simulink model "simulink_template_2_3_base"  (R2024b)
settings: Solver=FixedStepAuto  StartTime=0.0  StopTime=10.0  FixedStep=1e-3  RelTol=1e-3
values from neighbouring files (symbols this model uses):
  a = vc/Ta    (= 0.333333333333)    [fcn.m]    (also in part2.m = [xf,xi,kf*cos(thetaf)-3*xf, ki*cos(thetai)+3*xi ])
  b = [yf,yi,kf*sin(thetaf)-3*yf, ki*sin(thetai)+3*yi ]    [part2.m]
  qi = [-1; -1; pi/2]    [EX_opt_2_leo.m]    (also in part2.m = [xi;yi;thetai]; script_2_motion_planning.m)
settings Model: Creator=alber  LastModifiedBy=loren
settings RTWCC: GPUComputeCapability=3.5

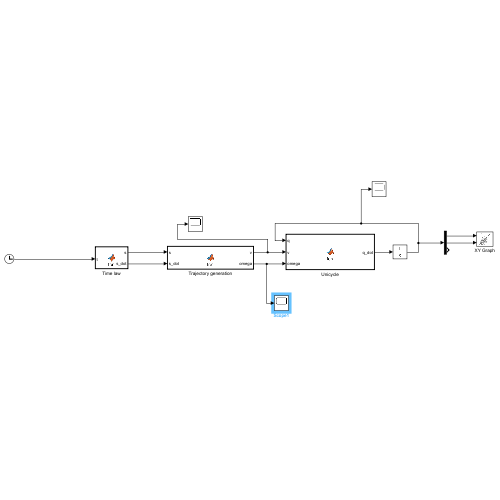
[thumbnail: Simulink's stored preview of the top-level diagram]
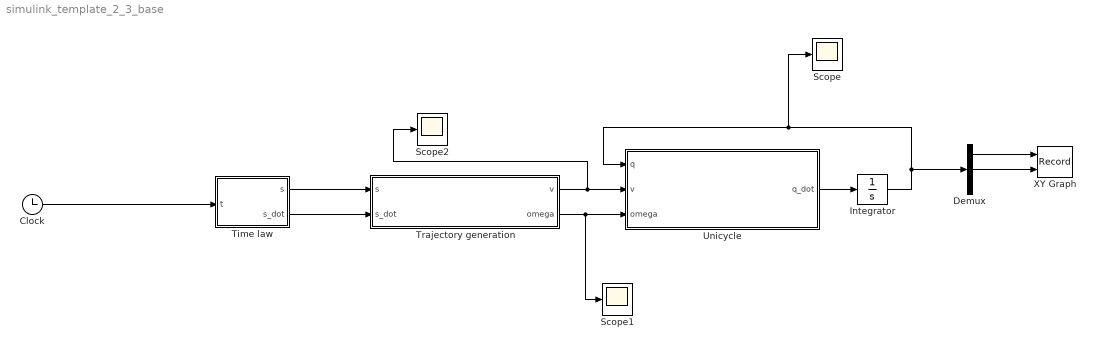
== system simulink_template_2_3_base ==
  Clock : Clock
  Demux : Demux  Outputs=3
  Integrator : Integrator  InitialCondition=qi
  Scope : Scope
  Scope1 : Scope
  Scope2 : Scope
  Time law : MATLAB Function  TreatAsAtomicUnit=on
  Trajectory generation : MATLAB Function  TreatAsAtomicUnit=on
  Unicycle : MATLAB Function  TreatAsAtomicUnit=on
  XY Graph : Record  FileSettingsInternal="{\"entries\":[{\"content\":{\"excelSettings\":{\"content\":{},\"type\":\"Streamout.ExcelSettings\"}},\"type\":\"Streamout.FileSettingStorage\",\"uuid\":\"\"}],\"packageUris\":[\"http:\\/\\/schema.mathworks.com\\/mf0\\/streamout_blocks\\/R2020a\"],\"version\":\"1.0\"}"  Layout=[1 1]  SignalsInternal="{\"entries\":[{\"content\":{\"signals\":[{\"content\":{\"blockPath\":[],\"dimensions\":[1,1],\"domain\":\"\",\"lineColor\":\"#a2142f\",\"lineWidth\":2,\"port\":1,\"sid\":[\"\"],\"signalID\":1,\"signalName\":\"Demux:1\"},\"type\":\"RecordBlkView.Signal\",\"uuid\":\"\"},{\"content\":{\"blockPath\":[],\"dimensions\":[1,1],\"domain\":\"\",\"lineColor\":\"#139fff\",\"plots\":[ 1 ],\"port\":2,\"sid\":[\"\"],\"signalID\":2,\"signalName\":\"Demux:2\"},\"type\":\"RecordBlkView.Signal\",\"uuid\":\"\"}]},\"type\":\"RecordBlkView.InputSignals\",\"uuid\":\"\"}],\"packageUris\":[\"http:\\/\\/schema.mathworks.com\\/mf0\\/streamout_blocks\\/R2020a\"],\"version\":\"1.0\"}"  VisualizationBindings="{\"xyplotplugin\":{\"info\":[{\"series\":[{\"bindingParametersList\":[{\"parameter\":\"Y-Axis\",\"signalID\":2,\"signalName\":\"Demux:2\"}],\"seriesID\":0}],\"subplotID\":1}]}}"  CompatibilityTag=XY
  wires:
  Clock/1 -> Time law/1(t)
  Time law/1(s) -> Trajectory generation/1(s)
  Time law/2(s_dot) -> Trajectory generation/2(s_dot)
  Trajectory generation/1(v) -> Scope2/1, Unicycle/2(v)
  Trajectory generation/2(omega) -> Scope1/1, Unicycle/3(omega)
  Unicycle/1(q_dot) -> Integrator/1
  Integrator/1 -> Scope/1, Unicycle/1(q), Demux/1
  Demux/1 -> XY Graph/1
  Demux/2 -> XY Graph/2

== matlab function simulink_template_2_3_base/Trajectory generation ==
  data: v output; s input; s_dot input; omega output; a parameter; b parameter
function [v, omega] = fcn(s, s_dot, a, b)
    % 1. Calcolo delle derivate spaziali prime (x' e y')
    % Basate sul polinomio cubico: y1(s) = a1*s^3 - a2*(s-1)^3 + a3*s^2*(s-1) + a4*s*(s-1)^2
    x_p = 3*a(1)*s^2 - a(2)*(3*s^2 - 6*s + 3) + a(3)*(3*s^2 - 2*s) + a(4)*(3*s^2 - 4*s + 1);
    y_p = 3*b(1)*s^2 - b(2)*(3*s^2 - 6*s + 3) + b(3)*(3*s^2 - 2*s) + b(4)*(3*s^2 - 4*s + 1);
    
    % 2. Calcolo delle derivate spaziali seconde (x'' e y'')
    x_pp = 6*a(1)*s - a(2)*(6*s - 6) + a(3)*(6*s - 2) + a(4)*(6*s - 4);
    y_pp = 6*b(1)*s - b(2)*(6*s - 6) + b(3)*(6*s - 2) + b(4)*(6*s - 4);
    
    % 3. Ingressi geometrici (tilde) assumendo marcia in avanti (k=0)
    v_tilde = sqrt(x_p^2 + y_p^2);
    
    % NOTA: Aggiungo 'eps' (un numero minuscolo) al denominatore per evitare 
    % che Simulink vada in crash per divisione per zero se il robot è fermo.
    omega_tilde = (x_p * y_pp - y_p * x_pp) / (x_p^2 + y_p^2 + eps);
    
    % 4. Ingressi fisici nel tempo (Moltiplicazione per s_dot)
    v = v_tilde * s_dot;
    omega = omega_tilde * s_dot;
end

== matlab function simulink_template_2_3_base/Time law ==
  data: t input; s output; s_dot output
function [s, s_dot] = fcn(t)
    % 1. Definizione dei parametri temporali (Puoi anche passarli come input del blocco)
    Ta = 1.0; % Tempo di accelerazione e decelerazione (Ta)
    Tc = 2.0; % Tempo a velocità costante (Tc)
    
    % 2. Calcolo di velocità e accelerazione come da slide
    vc = 1 / (Ta + Tc); % Velocità di crociera
    a = vc / Ta;        % Accelerazione
    
    % Inizializzazione delle variabili di uscita
    s = 0;
    s_dot = 0;
    
    % 3. Profilo di velocità trapezoidale (4 Fasi)
    if t < 0
        % Prima della partenza
        s = 0;
        s_dot = 0;
        
    elseif t < Ta
        % FASE 1: Accelerazione (0 <= t < Ta)
        s_dot = a * t;
        s = 0.5 * a * t^2;
        
    elseif t < (Ta + Tc)
        % FASE 2: Velocità costante (Ta <= t < Ta + Tc)
        s_dot = vc;
        % Spazio percorso alla fine della Fase 1 + spazio percorso a vel. costante
        s = (0.5 * a * Ta^2) + vc * (t - Ta);
        
    elseif t < (2*Ta + Tc)
        % FASE 3: Decelerazione (Ta + Tc <= t < 2Ta + Tc)
        dt = t - Ta - Tc; % Tempo trascorso dall'inizio della decelerazione
        s_dot = vc - a * dt;
        
        % Spazio totale alla fine della Fase 2
        s_fase2 = (0.5 * a * Ta^2) + vc * Tc;
        % Sommato allo spazio percorso durante la decelerazione
        s = s_fase2 + (vc * dt - 0.5 * a * dt^2);
        
    else
        % FASE 4: Arrivo (t >= 2Ta + Tc)
        % Assicura che si fermi esattamente a 1
        s = 1;
        s_dot = 0;
    end

end

== matlab function simulink_template_2_3_base/Unicycle ==
  data: q_dot output; q input; v input; omega input
function q_dot = fcn(q, v, omega)
    % Estrazione dell'angolo theta dal vettore di stato q
    % q(1) è la posizione x
    % q(2) è la posizione y
    % q(3) è l'orientamento theta
    theta = q(3);
    
    % Calcolo delle derivate dello stato (velocità lungo gli assi)
    x_dot = v * cos(theta);
    y_dot = v * sin(theta);
    theta_dot = omega;
    
    % Costruzione del vettore colonna di uscita q_dot
    q_dot = [x_dot; y_dot; theta_dot];
end
